simulink model "Cv_9_model"  (R2024a)
settings: Solver=FixedStepAuto  StartTime=0.0  StopTime=10  FixedStep=1e-6  RelTol=1e-3
values from neighbouring files (symbols this model uses):
  A = [0,     1,      0,      0,            0 ... (first row only)    [Cv_9_samostatna_prace.m]
  b = 0.5    [Cv_9_samostatna_prace.m]
  B = [0 0 0 0 1/L]'    [Cv_9_samostatna_prace.m]
  C = eye(5)    [Cv_9_samostatna_prace.m]
  D = zeros(5,1)    [Cv_9_samostatna_prace.m]
  i = 30    [Cv_9_samostatna_prace.m]
  J = J_r + J_b    (= 0.096)    [Cv_9_samostatna_prace.m]
  J_r = (1/3) * m_r * l^2    (= 0.06)    [Cv_9_samostatna_prace.m]
  k = 1480    [Cv_9_samostatna_prace.m]
  M = F * l    (= 3)    [Cv_9_samostatna_prace.m]
  omega = 0*0.5    (= 0)    [Cv_9_samostatna_prace.m]
settings Model: Creator=221208  LastModifiedBy=Miloš Uhlíř
settings ModelReferenceCC: EnableRefExpFcnMdlSchedulingChecks=on
settings RTWCC: GPUComputeCapability=3.5

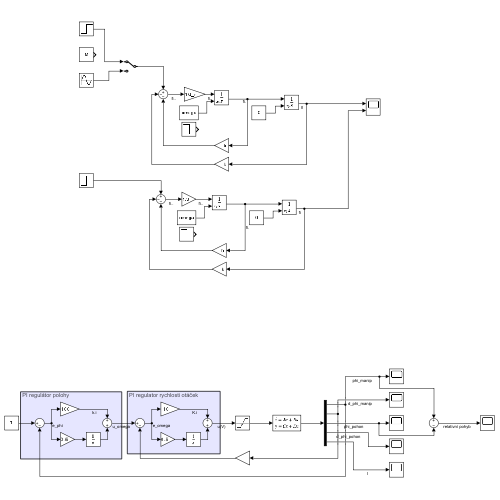
[thumbnail: Simulink's stored preview of the top-level diagram]
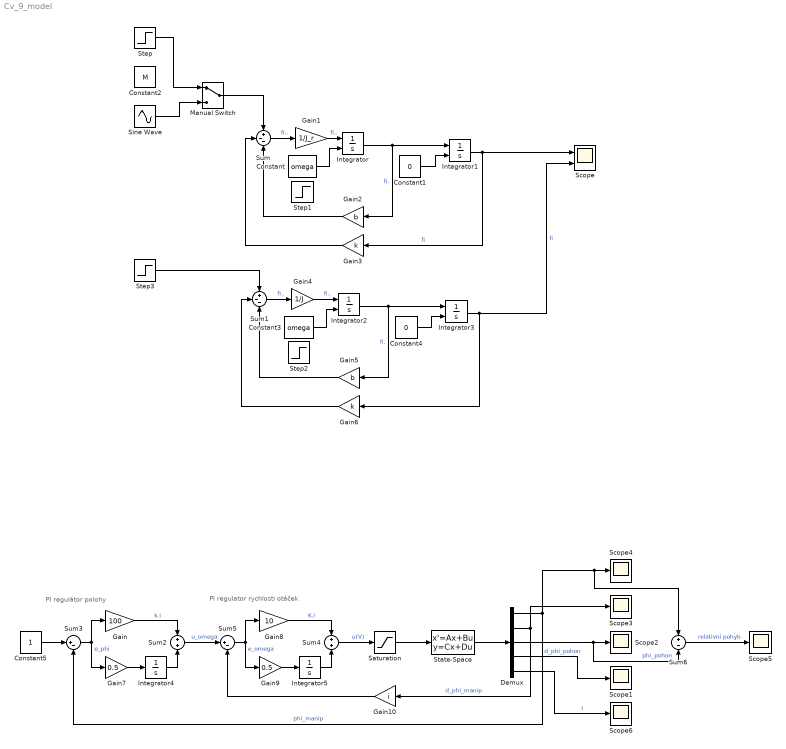
== system Cv_9_model ==
  note: PI regulator rychlosti otáček
  note: PI regulátor polohy
  Constant : Constant  Value=omega
  Constant1 : Constant  Value=0
  Constant2 : Constant  Value=M
  Constant3 : Constant  Value=omega
  Constant4 : Constant  Value=0
  Constant5 : Constant
  Demux : Demux  Outputs=5
  Gain : Gain  Gain=100
  Gain1 : Gain  Gain=1/J_r
  Gain10 : Gain  Gain=i
  Gain2 : Gain  Gain=b
  Gain3 : Gain  Gain=k
  Gain4 : Gain  Gain=1/J
  Gain5 : Gain  Gain=b
  Gain6 : Gain  Gain=k
  Gain7 : Gain  Gain=0.5
  Gain8 : Gain  Gain=10
  Gain9 : Gain  Gain=0.5
  Integrator{,1..3} (4 alike) : Integrator  InitialConditionSource=external
  Integrator4 : Integrator
  Integrator5 : Integrator
  Manual Switch : ManualSwitch
  Saturation : Saturate
  Scope : Scope  NumInputPorts=2
  Scope{1..6} (6 alike) : Scope
  Sine Wave : Sin  Amplitude=M  Frequency=10  SampleTime=0
  State-Space : StateSpace  A=A  B=B  C=C  D=D  InitialCondition=0
  Step : Step  Time=0  After=M  SampleTime=0
  Step1 : Step  Before=0.5  After=0  SampleTime=0
  Step2 : Step  Before=0.5  After=0  SampleTime=0
  Step3 : Step  Time=0  After=M  SampleTime=0
  Sum : Sum  Inputs=+--
  Sum1 : Sum  Inputs=+--
  Sum2 : Sum
  Sum3 : Sum  Inputs=|+-
  Sum4 : Sum
  Sum5 : Sum  Inputs=|+-
  Sum6 : Sum  Inputs=+-
  wires:
  Sum/1 -> Gain1/1  "fi.."
  Integrator/1 -> Integrator1/1, Gain2/1  "fi."
  Integrator1/1 -> Scope/1, Gain3/1  "fi"
  Gain2/1 -> Sum/3
  Gain3/1 -> Sum/2
  Gain1/1 -> Integrator/1  "fi.."
  Constant1/1 -> Integrator1/2
  Constant/1 -> Integrator/2
  Step/1 -> Manual Switch/1
  Sine Wave/1 -> Manual Switch/2
  Manual Switch/1 -> Sum/1
  Constant3/1 -> Integrator2/2
  Gain5/1 -> Sum1/3
  Gain4/1 -> Integrator2/1  "fi.."
  Integrator3/1 -> Scope/2, Gain6/1  "fi"
  Constant4/1 -> Integrator3/2
  Integrator2/1 -> Integrator3/1, Gain5/1  "fi."
  Sum1/1 -> Gain4/1  "fi.."
  Gain6/1 -> Sum1/2
  Step3/1 -> Sum1/1
  Gain7/1 -> Integrator4/1
  Sum3/1 -> Gain/1, Gain7/1  "e_phi"
  Integrator4/1 -> Sum2/2
  Gain/1 -> Sum2/1  "k.i"
  Constant5/1 -> Sum3/1
  Gain8/1 -> Sum4/1  "K.i"
  Integrator5/1 -> Sum4/2
  Sum5/1 -> Gain8/1, Gain9/1  "e_omega"
  Gain9/1 -> Integrator5/1
  Sum2/1 -> Sum5/1  "u_omega"
  Saturation/1 -> State-Space/1
  Sum4/1 -> Saturation/1  "u(V)"
  State-Space/1 -> Demux/1
  Demux/2 -> Gain10/1, Scope3/1  "d_phi_manip"
  Gain10/1 -> Sum5/2
  Demux/1 -> Scope4/1, Sum6/1, Sum3/2  "phi_manip"
  Demux/5 -> Scope6/1  "I"
  Demux/4 -> Scope1/1  "d_phi_pohon"
  Demux/3 -> Scope2/1, Sum6/2  "phi_pohon"
  Sum6/1 -> Scope5/1  "relativní pohyb"
